simulink model "TumorDetectionAlgorithm"  (R2023b)
settings: Solver=VariableStepAuto  StartTime=0.0  StopTime=10.0  RelTol=1e-3
libraries: simulink x10
settings Model: Creator=jsonm  LastModifiedBy=jsonm

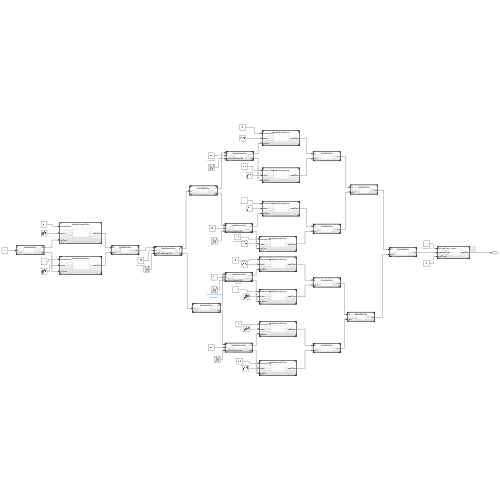
[thumbnail: Simulink's stored preview of the top-level diagram]
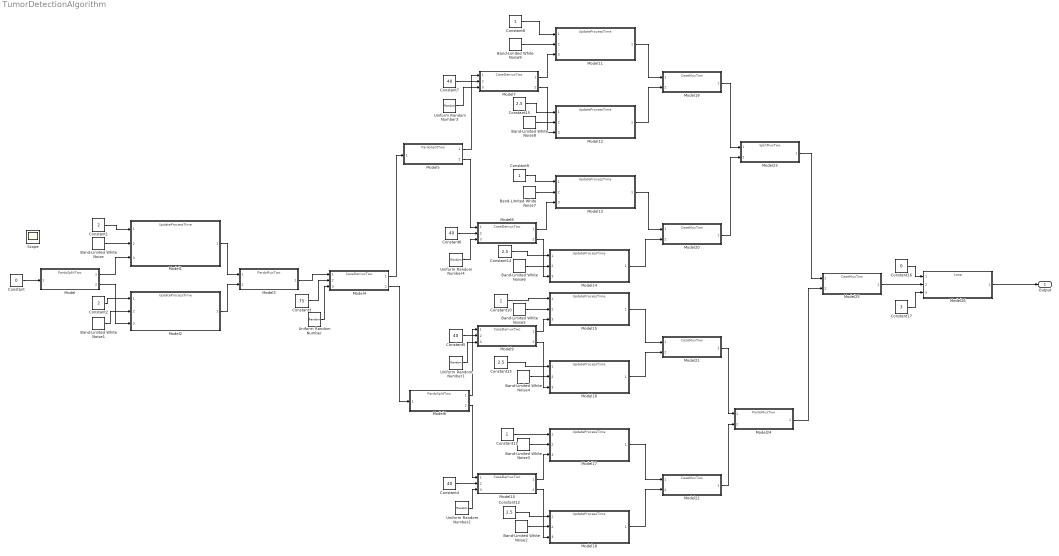
== system TumorDetectionAlgorithm ==
  Band-Limited White Noise{,1..9} (10 alike) : simulink/Sources/Band-Limited White Noise  Cov=[0.1]  Ts=0.1  seed=[23341]
  Constant : Constant  Value=0
  Constant1 : Constant  Value=2
  Constant{8..11} (4 alike) : Constant
  Constant{12..15} (4 alike) : Constant  Value=2.5
  Constant16 : Constant  Value=0
  Constant17 : Constant  Value=3
  Constant2 : Constant  Value=2
  Constant3 : Constant  Value=75
  Constant{4..7} (4 alike) : Constant  Value=40
  Model : ModelReference  ModelNameDialog=PardoSplitTwo.slx  SimulationMode=Normal  ModelReferenceVersion=1.3
  Model{1..2,11..18} (10 alike) : ModelReference  ModelNameDialog=UpdateProcessTime.slx  SimulationMode=Normal  ModelReferenceVersion=1.6
  Model{4,7..10} (5 alike) : ModelReference  ModelNameDialog=CaseDemuxTwo.slx  SimulationMode=Normal  ModelReferenceVersion=1.14
  Model{19..22,25} (5 alike) : ModelReference  ModelNameDialog=CaseMuxTwo.slx  SimulationMode=Normal  ModelReferenceVersion=1.6
  Model23 : ModelReference  ModelNameDialog=SplitMuxTwo.slx  SimulationMode=Normal  ModelReferenceVersion=1.4
  Model24 : ModelReference  ModelNameDialog=PardoMuxTwo.slx  SimulationMode=Normal  ModelReferenceVersion=1.5
  Model26 : ModelReference  ModelNameDialog=Loop.slx  SimulationMode=Normal  ModelReferenceVersion=1.1
  Model3 : ModelReference  ModelNameDialog=PardoMuxTwo.slx  SimulationMode=Normal  ModelReferenceVersion=1.5
  Model5 : ModelReference  ModelNameDialog=PardoSplitTwo.slx  SimulationMode=Normal  ModelReferenceVersion=1.3
  Model6 : ModelReference  ModelNameDialog=PardoSplitTwo.slx  SimulationMode=Normal  ModelReferenceVersion=1.3
  Uniform Random Number{,1..4} (5 alike) : UniformRandomNumber  Minimum=0  Maximum=100  SampleTime=0.1
  Output : Outport
  Scope : Scope
  wires:
  Model/1 -> Model1/3
  Model/2 -> Model2/3
  Model1/1 -> Model3/1
  Model2/1 -> Model3/2
  Constant/1 -> Model/1
  Model3/1 -> Model4/1
  Model4/1 -> Model5/1
  Model4/2 -> Model6/1
  Model26/1 -> Output/1
  Band-Limited White Noise/1 -> Model1/2
  Band-Limited White Noise1/1 -> Model2/2
  Constant1/1 -> Model1/1
  Constant2/1 -> Model2/1
  Uniform Random Number/1 -> Model4/3
  Constant3/1 -> Model4/2
  Model5/1 -> Model7/1
  Model5/2 -> Model8/1
  Model6/1 -> Model9/1
  Model6/2 -> Model10/1
  Uniform Random Number1/1 -> Model9/3
  Uniform Random Number2/1 -> Model10/3
  Uniform Random Number3/1 -> Model7/3
  Uniform Random Number4/1 -> Model8/3
  Constant4/1 -> Model10/2
  Constant5/1 -> Model9/2
  Constant6/1 -> Model8/2
  Constant7/1 -> Model7/2
  Model11/1 -> Model19/1
  Model12/1 -> Model19/2
  Model19/1 -> Model23/1
  Model13/1 -> Model20/1
  Model14/1 -> Model20/2
  Model20/1 -> Model23/2
  Model15/1 -> Model21/1
  Model16/1 -> Model21/2
  Model21/1 -> Model24/1
  Model17/1 -> Model22/1
  Model18/1 -> Model22/2
  Model22/1 -> Model24/2
  Model10/1 -> Model17/3
  Model10/2 -> Model18/3
  Model9/1 -> Model15/3
  Model9/2 -> Model16/3
  Model8/2 -> Model14/3
  Model8/1 -> Model13/3
  Model7/2 -> Model12/3
  Model7/1 -> Model11/3
  Band-Limited White Noise2/1 -> Model18/2
  Band-Limited White Noise3/1 -> Model17/2
  Band-Limited White Noise4/1 -> Model16/2
  Band-Limited White Noise5/1 -> Model15/2
  Band-Limited White Noise6/1 -> Model14/2
  Band-Limited White Noise7/1 -> Model13/2
  Band-Limited White Noise8/1 -> Model12/2
  Band-Limited White Noise9/1 -> Model11/2
  Constant8/1 -> Model11/1
  Constant9/1 -> Model13/1
  Constant10/1 -> Model15/1
  Constant11/1 -> Model17/1
  Constant12/1 -> Model18/1
  Constant13/1 -> Model16/1
  Constant14/1 -> Model14/1
  Constant15/1 -> Model12/1
  Model24/1 -> Model25/2
  Model23/1 -> Model25/1
  Model25/1 -> Model26/2
  Constant16/1 -> Model26/1
  Constant17/1 -> Model26/3
